simulink model "EV_Backward_Baseline"  (R2024b)
settings: Solver=FixedStepDiscrete  StartTime=EV_start  StopTime=EV_stop  FixedStep=EV_dt  RelTol=1e-3
values from neighbouring files (symbols this model uses):
  degradation_Crate = [0 0.5 1 2 3 4]    [init_ev_backward.m]    (also in initialize_model.m)
  degradation_rate = degradation_scale * [0 1 1.2 1.8 2.8 4.0]    [init_ev_backward.m]    (also in initialize_model.m = degradation_scale*degradation_relative_loss)
  ecvt_final_efficiency = EV_drive_eta    (= 0.96)    [init_ev_backward.m]    (also in initialize_model.m)
  ecvt_final_ratio = EV_final    (= 3)    [init_ev_backward.m]    (also in initialize_model.m)
  ecvt_parameters = [N_s N_r ecvt_motor1_Tmax ecvt_motor2_Tmax      ecvt_motor1_Pmax ecvt_motor2_Pmax motor1_wmax motor2_wmax      EV_motor_eta EV_regen_eta motor1_regen_fraction motor2_regen_fraction]    [init_ev_backward.m]    (also in initialize_model.m = [ecvt_parameters ecvt_strategy EV_voltage EV_resistance     )
  EV_Ah0 = 0    [initialize_model.m]
  EV_area = 2.2    [init_ev_backward.m]    (also in initialize_model.m)
  EV_capacity_Ah = 150    [init_ev_backward.m]    (also in initialize_model.m)
  EV_Cd = 0.29    [init_ev_backward.m]    (also in initialize_model.m)
  EV_Crr = 0.010    (= 0.01)    [init_ev_backward.m]    (also in initialize_model.m)
  EV_drive_eta = 0.96    [init_ev_backward.m]    (also in initialize_model.m)
  EV_dt = 0.1    [init_ev_backward.m]    (also in initialize_model.m)
  EV_final = 3    [init_ev_backward.m]    (also in initialize_model.m)
  EV_g = 9.81    [init_ev_backward.m]    (also in initialize_model.m)
  EV_gear = 3    [init_ev_backward.m]    (also in initialize_model.m)
  EV_grade = 0    [init_ev_backward.m]    (also in initialize_model.m)
  EV_mass = 1800    [init_ev_backward.m]    (also in initialize_model.m)
  EV_motor_eta = 0.92    [init_ev_backward.m]    (also in initialize_model.m)
  EV_radius = 0.31    [init_ev_backward.m]    (also in initialize_model.m)
  EV_regen_eta = 0.85    [init_ev_backward.m]    (also in initialize_model.m)
  EV_resistance = 0.08    [init_ev_backward.m]    (also in initialize_model.m)
  EV_rho = 1.225    [init_ev_backward.m]    (also in initialize_model.m)
  EV_SOC0 = 0.80    (= 0.8)    [init_ev_backward.m]    (also in initialize_model.m = 0.35)
  EV_SOH0 = 1.0    (= 1)    [init_ev_backward.m]    (also in initialize_model.m)
  EV_SOH_max = 1    [initialize_model.m]
  EV_SOH_min = 0    [initialize_model.m]
  EV_v0 = EV_speed(1)    [init_ev_backward.m]    (also in initialize_model.m)
  EV_voltage = 360    [init_ev_backward.m]    (also in initialize_model.m)
undefined symbols (not defined in the file or in its folder): DiscIntNeverNeededParam, ecvt_electrical_power, ecvt_operating_point
settings Model: Creator=menda  LastModifiedBy=menda

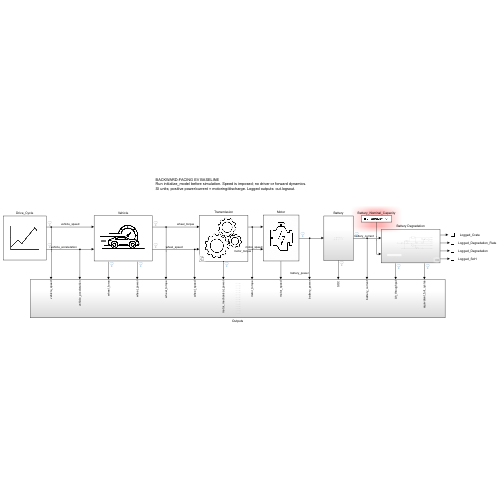
[thumbnail: Simulink's stored preview of the top-level diagram]
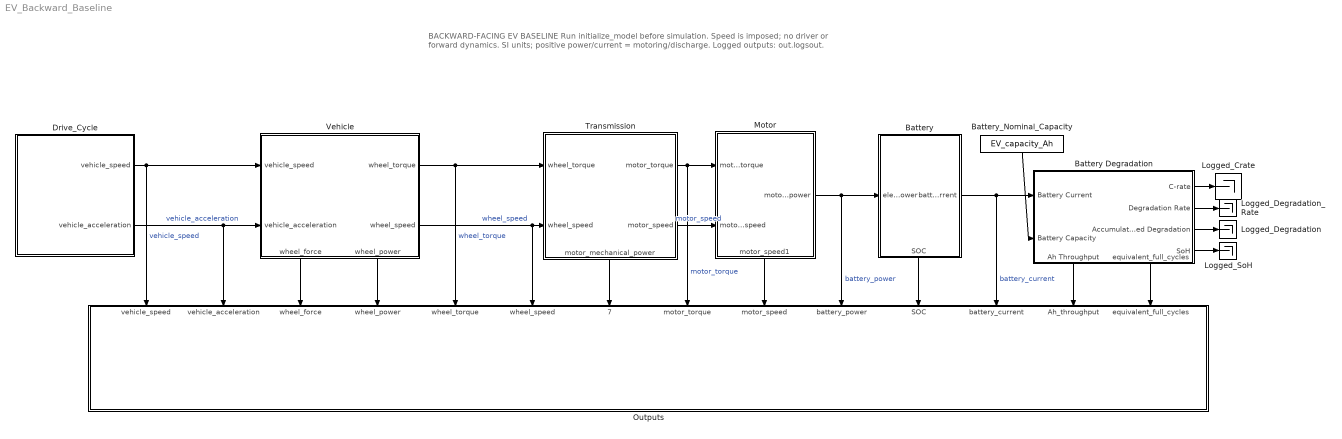
== system EV_Backward_Baseline ==
  note: BACKWARD-FACING EV BASELINE
      | Run initialize_model before simulation. Speed is imposed; no driver or forward dynamics.
      | SI units; positive power/current = motoring/discharge. Logged outputs: out.logsout.
  Battery : Subsystem  Description=Pbat=(Voc-R*I)*I; I=2*Pbat/(Voc+sqrt(Voc^2-4*R*Pbat)); dSOC/dt=-I/(3600*capacity_Ah). Positive I discharges. Assertions stop for infeasible power or SOC outside [0,1]. abs under sqrt only guards evaluation before the power assertion; it does not authorize infeasible demands.
      settings: PortSchema="{\"entries\":[{\"content\":{\"sides\":[{\"content\":{\"connectorIds\":[\"In1\"]},\"type\":\"ConnectorPlacement.EquallySpacedRectSide\",\"uuid\":\"e30f2f7f-bb89-4748-9a65-d09dfa466cc4\"},{\"content\":{\"connectorIds\":[\"Out1\"],\"side\":\"RIGHT\"},\"type\":\"ConnectorPlacement.EquallySpacedRectSide\",\"uuid\":\"7aa5349f-4bb4-43b6-83e0-f5db2de7542c\"},{\"content\":{\"side\":\"TOP\"},\"type\":\"ConnectorPlacement.EquallySpacedRectSide\",\"uuid\":\"10c9eaa9-2802-435c-9c7b-7eaef7f59c40\"},{\"content\":{\"connectorIds\":[\"Out2\"],\"side\":\"BOTTOM\"},\"type\":\"ConnectorPlacement.EquallySpacedRectSide\",\"uuid\":\"ef51e7df-83e2-4289-b7c3-b47825779f33\"}]},\"type\":\"ConnectorPlacement.EquallySpacedConnector\",\"uuid\":\"367388d2-e83d-4c8a-b099-5ce472d0570c\"}],\"packageUris\":[\"http://schema.mathworks.com/mf0/Connector/R2020b\"],\"version\":\"1.0\"}"
  Battery Degradation : Subsystem  Description=C=abs(I)/Qnom; k=f(C) [1/Ah], linear with endpoint clipping. dD/dt=k*abs(I)/3600 [1/s]; D0=1-EV_SOH0. SoH=sat(1-D,0,1). No feedback to SOC or capacity.
      settings: PortSchema="{\"entries\":[{\"content\":{\"sides\":[{\"content\":{\"connectorIds\":[\"In1\",\"In2\"]},\"type\":\"ConnectorPlacement.EquallySpacedRectSide\",\"uuid\":\"b05f624b-af73-4004-9694-629fd8fb527f\"},{\"content\":{\"connectorIds\":[\"Out1\",\"Out2\",\"Out3\",\"Out4\"],\"side\":\"RIGHT\"},\"type\":\"ConnectorPlacement.EquallySpacedRectSide\",\"uuid\":\"830d9b11-fa0e-4f63-a09e-821a7b3aefa4\"},{\"content\":{\"side\":\"TOP\"},\"type\":\"ConnectorPlacement.EquallySpacedRectSide\",\"uuid\":\"ac9d2d09-daf1-45c6-b99a-e7004515f525\"},{\"content\":{\"connectorIds\":[\"Out5\",\"Out6\"],\"side\":\"BOTTOM\"},\"type\":\"ConnectorPlacement.EquallySpacedRectSide\",\"uuid\":\"9e730963-03db-478a-aca3-248f9a9dc559\"}]},\"type\":\"ConnectorPlacement.EquallySpacedConnector\",\"uuid\":\"6a4c7b58-1cfe-457b-b589-490fcd40ae9b\"}],\"packageUris\":[\"http://schema.mathworks.com/mf0/Connector/R2020b\"],\"version\":\"1.0\"}"
  Battery_Nominal_Capacity : Constant  Value=EV_capacity_Ah
  Drive_Cycle : Subsystem  Description=Prescribed sampled speed [m/s]. a[k]=(v[k]-v[k-1])/EV_dt [m/s^2]. Initial acceleration is zero.
      mask Display: image('images/speedProfile.png');
  Logged_Crate : Terminator
  Logged_Degradation : Terminator
  Logged_Degradation_Rate : Terminator
  Logged_SoH : Terminator
  Motor : Subsystem  Description=Pmech=T*omega; Pelec=Pmech/eta_motor when Pmech>=0, otherwise Pmech*eta_regen. Positive means motoring. Torque and speed are imposed by Transmission and logged at its outputs.
      settings: PortSchema="{\"entries\":[{\"content\":{\"sides\":[{\"content\":{\"connectorIds\":[\"In1\",\"In2\"]},\"type\":\"ConnectorPlacement.EquallySpacedRectSide\",\"uuid\":\"49c52859-d992-4436-ae70-9d5acb989b00\"},{\"content\":{\"connectorIds\":[\"Out1\"],\"side\":\"RIGHT\"},\"type\":\"ConnectorPlacement.EquallySpacedRectSide\",\"uuid\":\"a77a678a-5372-480a-805a-36d1e2fecae4\"},{\"content\":{\"side\":\"TOP\"},\"type\":\"ConnectorPlacement.EquallySpacedRectSide\",\"uuid\":\"187b8372-9e3a-4a7e-b220-549ea4957a3e\"},{\"content\":{\"connectorIds\":[\"Out2\"],\"side\":\"BOTTOM\"},\"type\":\"ConnectorPlacement.EquallySpacedRectSide\",\"uuid\":\"92a127f9-6f51-4bd3-badd-4b9089e059fd\"}]},\"type\":\"ConnectorPlacement.EquallySpacedConnector\",\"uuid\":\"4c2fc29c-556e-423a-96d4-0ac59323ac06\"}],\"packageUris\":[\"http://schema.mathworks.com/mf0/Connector/R2020b\"],\"version\":\"1.0\"}"
      mask Display: image('images/engine2.jpg');
  Outputs : Subsystem
  Transmission : Subsystem  Description=Variant powertrain topology. EV_topology=1 selects single motor, fixed gear and differential. Match port names in future choices.  Variant=on
      settings: PortSchema="{\"entries\":[{\"content\":{\"sides\":[{\"content\":{\"connectorIds\":[\"In1\",\"In2\"]},\"type\":\"ConnectorPlacement.EquallySpacedRectSide\",\"uuid\":\"907b9752-0237-4bf5-b44c-0c58cc455c3d\"},{\"content\":{\"connectorIds\":[\"Out1\",\"Out2\"],\"side\":\"RIGHT\"},\"type\":\"ConnectorPlacement.EquallySpacedRectSide\",\"uuid\":\"60baf348-a017-4c22-82d9-e85b283ea42b\"},{\"content\":{\"side\":\"TOP\"},\"type\":\"ConnectorPlacement.EquallySpacedRectSide\",\"uuid\":\"1e1150ea-72dd-48d2-abb5-aeef63cf3690\"},{\"content\":{\"connectorIds\":[\"Out3\"],\"side\":\"BOTTOM\"},\"type\":\"ConnectorPlacement.EquallySpacedRectSide\",\"uuid\":\"c29cbbf6-43d5-4701-ab56-40ad23203659\"}]},\"type\":\"ConnectorPlacement.EquallySpacedConnector\",\"uuid\":\"b8b54c79-4f22-4cf5-bff2-51665ec3e128\"}],\"packageUris\":[\"http://schema.mathworks.com/mf0/Connector/R2020b\"],\"version\":\"1.0\"}"
      mask Display: image('images/Gearbox.png');
  Vehicle : Subsystem  Description=F=m*a+0.5*rho*Cd*A*v*abs(v)+Crr*m*g*cos(grade)*sign(v)+m*g*sin(grade). T=F*r; omega=v/r; P=T*omega. SI units.
      settings: PortSchema="{\"entries\":[{\"content\":{\"sides\":[{\"content\":{\"connectorIds\":[\"In1\",\"In2\"]},\"type\":\"ConnectorPlacement.EquallySpacedRectSide\",\"uuid\":\"b24511cd-7d01-487c-854b-51850ccf7238\"},{\"content\":{\"connectorIds\":[\"Out1\",\"Out2\"],\"side\":\"RIGHT\"},\"type\":\"ConnectorPlacement.EquallySpacedRectSide\",\"uuid\":\"d60f9975-1cca-4220-8342-8a527ad4bc8f\"},{\"content\":{\"side\":\"TOP\"},\"type\":\"ConnectorPlacement.EquallySpacedRectSide\",\"uuid\":\"ffffd604-d748-4b68-bba9-21435e47b16e\"},{\"content\":{\"connectorIds\":[\"Out3\",\"Out4\"],\"side\":\"BOTTOM\"},\"type\":\"ConnectorPlacement.EquallySpacedRectSide\",\"uuid\":\"c964c0b3-1bf1-4a71-99c2-52acac1d6e4c\"}]},\"type\":\"ConnectorPlacement.EquallySpacedConnector\",\"uuid\":\"2b03c9da-f0d0-45d9-9588-bb20003291c2\"}],\"packageUris\":[\"http://schema.mathworks.com/mf0/Connector/R2020b\"],\"version\":\"1.0\"}"
      mask Display: image('images/Dynamics.png');
  wires:
  Vehicle/1(wheel_torque) -> Outputs/5(wheel_torque), Transmission/1(wheel_torque)  "wheel_torque"
  Drive_Cycle/1(vehicle_speed) -> Outputs/1(vehicle_speed), Vehicle/1(vehicle_speed)  "vehicle_speed"
  Drive_Cycle/2(vehicle_acceleration) -> Outputs/2(vehicle_acceleration), Vehicle/2(vehicle_acceleration)  "vehicle_acceleration"
  Vehicle/2(wheel_speed) -> Outputs/6(wheel_speed), Transmission/2(wheel_speed)  "wheel_speed"
  Battery/1(battery_current) -> Outputs/12(battery_current), Battery Degradation/1(Battery Current)  "battery_current"
  Vehicle/3(wheel_force) -> Outputs/3(wheel_force)
  Vehicle/4(wheel_power) -> Outputs/4(wheel_power)
  Motor/1(motor_electrical_power) -> Outputs/10(battery_power), Battery/1(electrical_power)  "battery_power"
  Battery/2(SOC) -> Outputs/11(SOC)
  Battery Degradation/5(Ah Throughput) -> Outputs/13(Ah_throughput)
  Battery Degradation/6(equivalent_full_cycles) -> Outputs/14(equivalent_full_cycles)
  Transmission/3(motor_mechanical_power) -> Outputs/7(motor_mechanical_power)
  Transmission/1(motor_torque) -> Outputs/8(motor_torque), Motor/1(motor_torque)  "motor_torque"
  Transmission/2(motor_speed) -> Motor/2(motor_speed)  "motor_speed"
  Battery_Nominal_Capacity/1 -> Battery Degradation/2(Battery Capacity)
  Battery Degradation/1(C-rate) -> Logged_Crate/1
  Battery Degradation/2(Degradation Rate) -> Logged_Degradation_Rate/1
  Battery Degradation/3(Accumulated Degradation) -> Logged_Degradation/1
  Battery Degradation/4(SoH) -> Logged_SoH/1
  Motor/2(motor_speed1) -> Outputs/9(motor_speed)

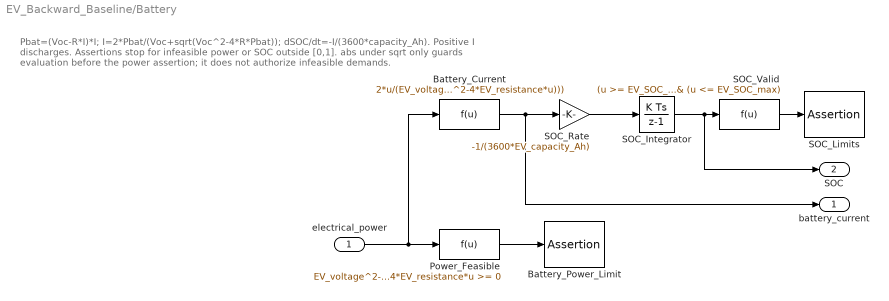
== system EV_Backward_Baseline/Battery ==
  note: Pbat=(Voc-R*I)*I; I=2*Pbat/(Voc+sqrt(Voc^2-4*R*Pbat)); dSOC/dt=-I/(3600*capacity_Ah). Positive I discharges. Assertions stop for infeasible power or SOC outside [0,1]. abs under sqrt only guards evaluation before the power assertion; it does not authorize infeasible demands.
  electrical_power : Inport
  Battery_Current : Fcn  Expr=2*u/(EV_voltage+sqrt(abs(EV_voltage^2-4*EV_resistance*u)))
  Battery_Power_Limit : Assertion
  Power_Feasible : Fcn  Expr=EV_voltage^2-4*EV_resistance*u >= 0
  SOC_Integrator : DiscreteIntegrator  InitialCondition=EV_SOC0  SampleTime=EV_dt  ICPrevOutput=DiscIntNeverNeededParam  ICPrevScaledInput=DiscIntNeverNeededParam
  SOC_Limits : Assertion
  SOC_Rate : Gain  Gain=-1/(3600*EV_capacity_Ah)
  SOC_Valid : Fcn  Expr=(u >= EV_SOC_min) && (u <= EV_SOC_max)
  battery_current : Outport
  SOC : Outport  Port=2
  wires:
  SOC_Valid/1 -> SOC_Limits/1
  SOC_Integrator/1 -> SOC/1, SOC_Valid/1
  SOC_Rate/1 -> SOC_Integrator/1
  Battery_Current/1 -> battery_current/1, SOC_Rate/1
  Power_Feasible/1 -> Battery_Power_Limit/1
  electrical_power/1 -> Battery_Current/1, Power_Feasible/1

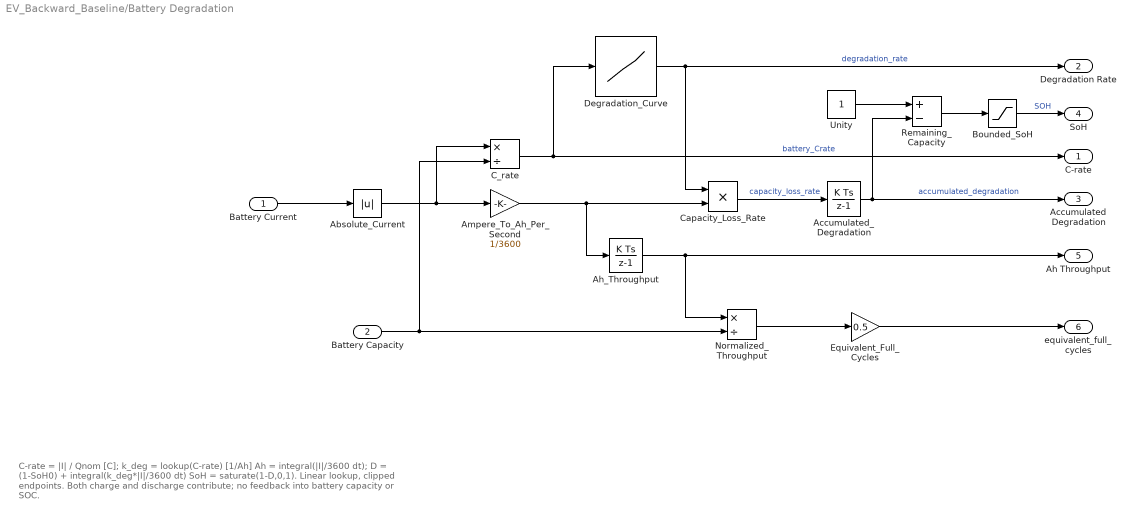
== system EV_Backward_Baseline/Battery Degradation ==
  note: C-rate = |I| / Qnom [C]; k_deg = lookup(C-rate) [1/Ah]
      | Ah = integral(|I|/3600 dt); D = (1-SoH0) + integral(k_deg*|I|/3600 dt)
      | SoH = saturate(1-D,0,1). Linear lookup, clipped endpoints.
      | Both charge and discharge contribute; no feedback into battery capacity or SOC.
  Battery Current : Inport
  Battery Capacity : Inport  Port=2
  Absolute_Current : Abs  SaturateOnIntegerOverflow=off
  Accumulated_Degradation : DiscreteIntegrator  InitialCondition=1-EV_SOH0  SampleTime=EV_dt  ICPrevOutput=DiscIntNeverNeededParam  ICPrevScaledInput=DiscIntNeverNeededParam
  Ah_Throughput : DiscreteIntegrator  InitialCondition=EV_Ah0  SampleTime=EV_dt  ICPrevOutput=DiscIntNeverNeededParam  ICPrevScaledInput=DiscIntNeverNeededParam
  Ampere_To_Ah_Per_Second : Gain  Gain=1/3600
  Bounded_SoH : Saturate  UpperLimit=EV_SOH_max  LowerLimit=EV_SOH_min
  C_rate : Product  Inputs=*/
  Capacity_Loss_Rate : Product  Inputs=**
  Degradation_Curve : Lookup_n-D  NumberOfTableDimensions=1  BreakpointsForDimension1=degradation_Crate  Table=degradation_rate  ExtrapMethod=Clip  InternalRulePriority=Speed  RndMeth=Simplest
  Equivalent_Full_Cycles : Gain  Gain=0.5
  Normalized_Throughput : Product  Inputs=*/
  Remaining_Capacity : Sum  Inputs=+-
  Unity : Constant
  C-rate : Outport
  Degradation Rate : Outport  Port=2
  Accumulated Degradation : Outport  Port=3
  SoH : Outport  Port=4
  Ah Throughput : Outport  Port=5
  equivalent_full_cycles : Outport  Port=6
  wires:
  Normalized_Throughput/1 -> Equivalent_Full_Cycles/1
  Bounded_SoH/1 -> SoH/1  "SOH"
  Remaining_Capacity/1 -> Bounded_SoH/1
  Unity/1 -> Remaining_Capacity/1
  Accumulated_Degradation/1 -> Accumulated Degradation/1, Remaining_Capacity/2  "accumulated_degradation"
  Capacity_Loss_Rate/1 -> Accumulated_Degradation/1  "capacity_loss_rate"
  Degradation_Curve/1 -> Capacity_Loss_Rate/1, Degradation Rate/1  "degradation_rate"
  C_rate/1 -> Degradation_Curve/1, C-rate/1  "battery_Crate"
  Battery Capacity/1 -> C_rate/2, Normalized_Throughput/2
  Absolute_Current/1 -> C_rate/1, Ampere_To_Ah_Per_Second/1
  Ampere_To_Ah_Per_Second/1 -> Ah_Throughput/1, Capacity_Loss_Rate/2
  Ah_Throughput/1 -> Ah Throughput/1, Normalized_Throughput/1
  Equivalent_Full_Cycles/1 -> equivalent_full_cycles/1
  Battery Current/1 -> Absolute_Current/1

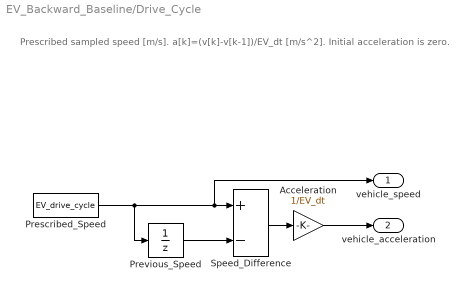
== system EV_Backward_Baseline/Drive_Cycle ==
  note: Prescribed sampled speed [m/s]. a[k]=(v[k]-v[k-1])/EV_dt [m/s^2]. Initial acceleration is zero.
  Acceleration : Gain  Gain=1/EV_dt
  Prescribed_Speed : FromWorkspace  VariableName=EV_drive_cycle  SampleTime=EV_dt
  Previous_Speed : UnitDelay  InitialCondition=EV_v0  SampleTime=EV_dt  HasFrameUpgradeWarning=on
  Speed_Difference : Sum  Inputs=+-
  vehicle_speed : Outport
  vehicle_acceleration : Outport  Port=2
  wires:
  Acceleration/1 -> vehicle_acceleration/1
  Speed_Difference/1 -> Acceleration/1
  Previous_Speed/1 -> Speed_Difference/2
  Prescribed_Speed/1 -> vehicle_speed/1, Speed_Difference/1, Previous_Speed/1

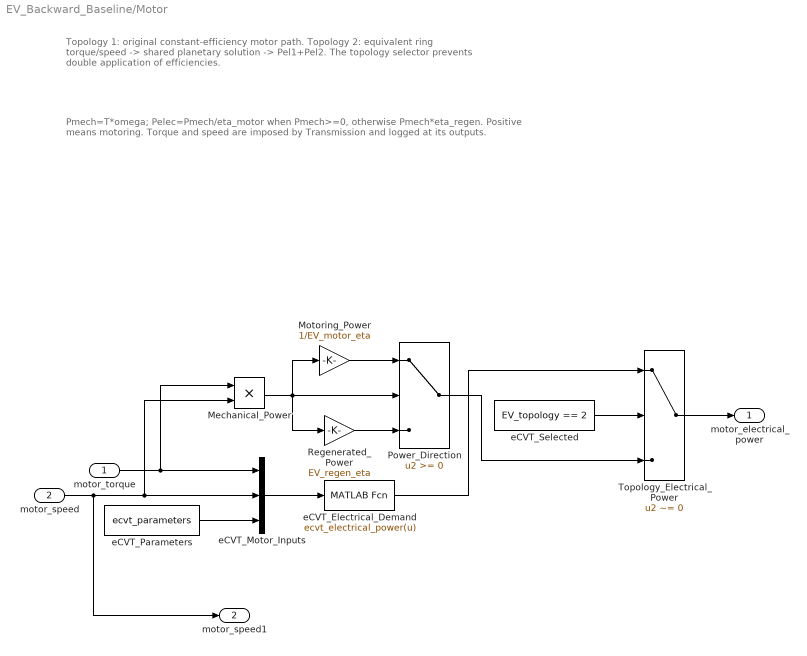
== system EV_Backward_Baseline/Motor ==
  note: Pmech=T*omega; Pelec=Pmech/eta_motor when Pmech>=0, otherwise Pmech*eta_regen. Positive means motoring. Torque and speed are imposed by Transmission and logged at its outputs.
  note: Topology 1: original constant-efficiency motor path.
      | Topology 2: equivalent ring torque/speed -> shared planetary solution -> Pel1+Pel2.
      | The topology selector prevents double application of efficiencies.
  motor_torque : Inport
  motor_speed : Inport  Port=2
  Mechanical_Power : Product
  Motoring_Power : Gain  Gain=1/EV_motor_eta
  Power_Direction : Switch  SaturateOnIntegerOverflow=off  InputSameDT=off
  Regenerated_Power : Gain  Gain=EV_regen_eta
  Topology_Electrical_Power : Switch  Criteria=u2 ~= 0  SaturateOnIntegerOverflow=off  InputSameDT=off
  eCVT_Electrical_Demand : MATLABFcn  MATLABFcn=ecvt_electrical_power(u)  OutputDimensions=1
  eCVT_Motor_Inputs : Mux  Inputs=3
  eCVT_Parameters : Constant  Value=ecvt_parameters
  eCVT_Selected : Constant  Value=EV_topology == 2
  motor_electrical_power : Outport
  motor_speed1 : Outport  Port=2
  wires:
  motor_torque/1 -> Mechanical_Power/1, eCVT_Motor_Inputs/1
  motor_speed/1 -> motor_speed1/1, eCVT_Motor_Inputs/2, Mechanical_Power/2
  Mechanical_Power/1 -> Regenerated_Power/1, Motoring_Power/1, Power_Direction/2
  Motoring_Power/1 -> Power_Direction/1
  Regenerated_Power/1 -> Power_Direction/3
  Topology_Electrical_Power/1 -> motor_electrical_power/1
  eCVT_Selected/1 -> Topology_Electrical_Power/2
  eCVT_Electrical_Demand/1 -> Topology_Electrical_Power/1
  Power_Direction/1 -> Topology_Electrical_Power/3
  eCVT_Parameters/1 -> eCVT_Motor_Inputs/3
  eCVT_Motor_Inputs/1 -> eCVT_Electrical_Demand/1

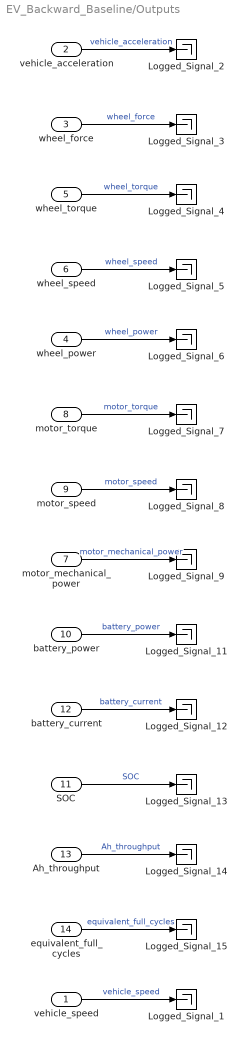
== system EV_Backward_Baseline/Outputs ==
  vehicle_speed : Inport
  vehicle_acceleration : Inport  Port=2
  wheel_force : Inport  Port=3
  wheel_power : Inport  Port=4
  wheel_torque : Inport  Port=5
  wheel_speed : Inport  Port=6
  motor_mechanical_power : Inport  Port=7
  motor_torque : Inport  Port=8
  motor_speed : Inport  Port=9
  battery_power : Inport  Port=10
  SOC : Inport  Port=11
  battery_current : Inport  Port=12
  Ah_throughput : Inport  Port=13
  equivalent_full_cycles : Inport  Port=14
  Logged_Signal_{1..9,11..15} (14 alike) : Terminator
  wires:
  vehicle_speed/1 -> Logged_Signal_1/1  "vehicle_speed"
  vehicle_acceleration/1 -> Logged_Signal_2/1  "vehicle_acceleration"
  wheel_force/1 -> Logged_Signal_3/1  "wheel_force"
  wheel_torque/1 -> Logged_Signal_4/1  "wheel_torque"
  wheel_speed/1 -> Logged_Signal_5/1  "wheel_speed"
  wheel_power/1 -> Logged_Signal_6/1  "wheel_power"
  motor_torque/1 -> Logged_Signal_7/1  "motor_torque"
  motor_speed/1 -> Logged_Signal_8/1  "motor_speed"
  motor_mechanical_power/1 -> Logged_Signal_9/1  "motor_mechanical_power"
  battery_power/1 -> Logged_Signal_11/1  "battery_power"
  battery_current/1 -> Logged_Signal_12/1  "battery_current"
  SOC/1 -> Logged_Signal_13/1  "SOC"
  Ah_throughput/1 -> Logged_Signal_14/1  "Ah_throughput"
  equivalent_full_cycles/1 -> Logged_Signal_15/1  "equivalent_full_cycles"

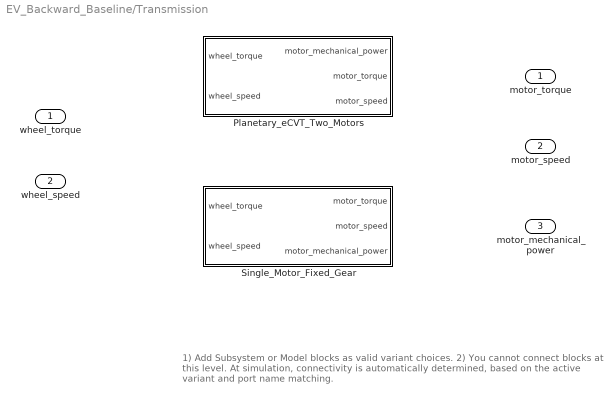
== system EV_Backward_Baseline/Transmission ==
  note: 1) Add Subsystem or Model blocks as valid variant choices.
      | 2) You cannot connect blocks at this level. At simulation, connectivity is automatically
      | determined, based on the active variant and port name matching.
  wheel_torque : Inport
  wheel_speed : Inport  Port=2
  Planetary_eCVT_Two_Motors : Subsystem  Description=Ideal planetary: M1 sun, M2 carrier, output ring. Scalar outputs are equivalent ring mechanical power/torque/speed. See README_eCVT.md.  VariantControl=EV_topology == 2
  Single_Motor_Fixed_Gear : Subsystem  Description=ratio=EV_gear*EV_final; omega_m=ratio*omega_w. T_m=T_w/(ratio*eta_d) for motoring, T_w*eta_d/ratio for regeneration. Combined gear/differential losses; no shaft inertia.  VariantControl=EV_topology == 1
  motor_torque : Outport
  motor_speed : Outport  Port=2
  motor_mechanical_power : Outport  Port=3

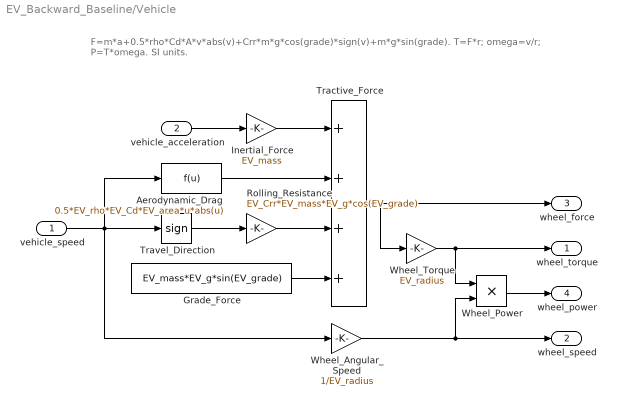
== system EV_Backward_Baseline/Vehicle ==
  note: F=m*a+0.5*rho*Cd*A*v*abs(v)+Crr*m*g*cos(grade)*sign(v)+m*g*sin(grade). T=F*r; omega=v/r; P=T*omega. SI units.
  vehicle_speed : Inport
  vehicle_acceleration : Inport  Port=2
  Aerodynamic_Drag : Fcn  Expr=0.5*EV_rho*EV_Cd*EV_area*u*abs(u)
  Grade_Force : Constant  Value=EV_mass*EV_g*sin(EV_grade)
  Inertial_Force : Gain  Gain=EV_mass
  Rolling_Resistance : Gain  Gain=EV_Crr*EV_mass*EV_g*cos(EV_grade)
  Tractive_Force : Sum  Inputs=++++
  Travel_Direction : Signum
  Wheel_Angular_Speed : Gain  Gain=1/EV_radius
  Wheel_Power : Product
  Wheel_Torque : Gain  Gain=EV_radius
  wheel_torque : Outport
  wheel_speed : Outport  Port=2
  wheel_force : Outport  Port=3
  wheel_power : Outport  Port=4
  wires:
  Wheel_Power/1 -> wheel_power/1
  Wheel_Angular_Speed/1 -> wheel_speed/1, Wheel_Power/2
  Wheel_Torque/1 -> Wheel_Power/1, wheel_torque/1
  Tractive_Force/1 -> wheel_force/1, Wheel_Torque/1
  Grade_Force/1 -> Tractive_Force/4
  Rolling_Resistance/1 -> Tractive_Force/3
  Aerodynamic_Drag/1 -> Tractive_Force/2
  Inertial_Force/1 -> Tractive_Force/1
  Travel_Direction/1 -> Rolling_Resistance/1
  vehicle_acceleration/1 -> Inertial_Force/1
  vehicle_speed/1 -> Wheel_Angular_Speed/1, Aerodynamic_Drag/1, Travel_Direction/1

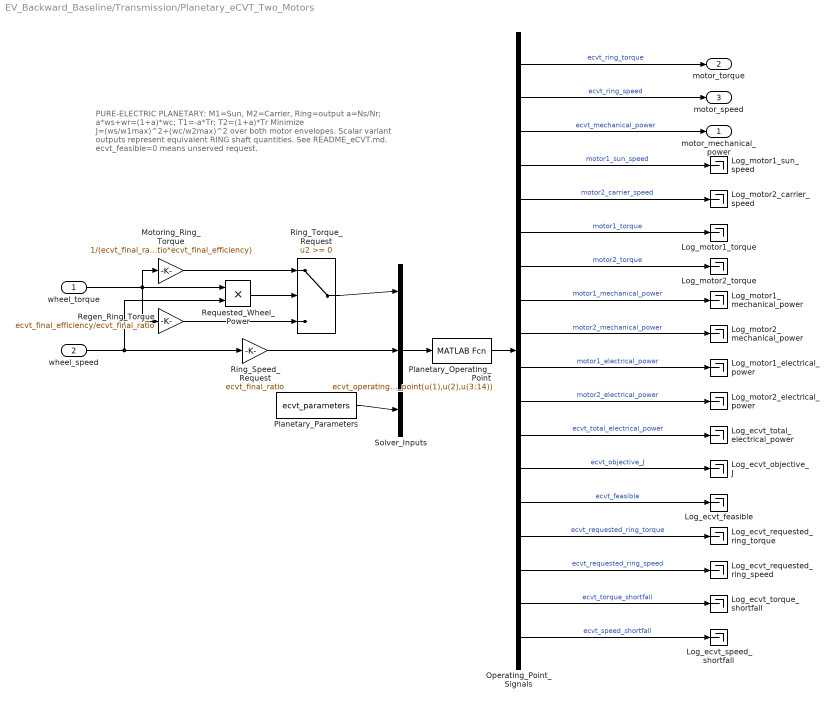
== system EV_Backward_Baseline/Transmission/Planetary_eCVT_Two_Motors ==
  note: PURE-ELECTRIC PLANETARY: M1=Sun, M2=Carrier, Ring=output
      | a=Ns/Nr; a*ws+wr=(1+a)*wc; T1=-a*Tr; T2=(1+a)*Tr
      | Minimize J=(ws/w1max)^2+(wc/w2max)^2 over both motor envelopes.
      | Scalar variant outputs represent equivalent RING shaft quantities.
      | See README_eCVT.md. ecvt_feasible=0 means unserved request.
  wheel_torque : Inport
  wheel_speed : Inport  Port=2
  Log_ecvt_feasible : Terminator
  Log_ecvt_objective_J : Terminator
  Log_ecvt_requested_ring_speed : Terminator
  Log_ecvt_requested_ring_torque : Terminator
  Log_ecvt_speed_shortfall : Terminator
  Log_ecvt_torque_shortfall : Terminator
  Log_ecvt_total_electrical_power : Terminator
  Log_motor1_electrical_power : Terminator
  Log_motor1_mechanical_power : Terminator
  Log_motor1_sun_speed : Terminator
  Log_motor1_torque : Terminator
  Log_motor2_carrier_speed : Terminator
  Log_motor2_electrical_power : Terminator
  Log_motor2_mechanical_power : Terminator
  Log_motor2_torque : Terminator
  Motoring_Ring_Torque : Gain  Gain=1/(ecvt_final_ratio*ecvt_final_efficiency)
  Operating_Point_Signals : Demux  Outputs=18
  Planetary_Operating_Point : MATLABFcn  MATLABFcn=ecvt_operating_point(u(1),u(2),u(3:14))  OutputDimensions=18
  Planetary_Parameters : Constant  Value=ecvt_parameters
  Regen_Ring_Torque : Gain  Gain=ecvt_final_efficiency/ecvt_final_ratio
  Requested_Wheel_Power : Product  Inputs=**
  Ring_Speed_Request : Gain  Gain=ecvt_final_ratio
  Ring_Torque_Request : Switch  SaturateOnIntegerOverflow=off  InputSameDT=off
  Solver_Inputs : Mux  Inputs=3
  motor_mechanical_power : Outport
  motor_torque : Outport  Port=2
  motor_speed : Outport  Port=3
  wires:
  wheel_torque/1 -> Regen_Ring_Torque/1, Motoring_Ring_Torque/1, Requested_Wheel_Power/1
  wheel_speed/1 -> Requested_Wheel_Power/2, Ring_Speed_Request/1
  Motoring_Ring_Torque/1 -> Ring_Torque_Request/1
  Requested_Wheel_Power/1 -> Ring_Torque_Request/2
  Regen_Ring_Torque/1 -> Ring_Torque_Request/3
  Operating_Point_Signals/4 -> Log_motor1_sun_speed/1  "motor1_sun_speed"
  Operating_Point_Signals/5 -> Log_motor2_carrier_speed/1  "motor2_carrier_speed"
  Operating_Point_Signals/6 -> Log_motor1_torque/1  "motor1_torque"
  Operating_Point_Signals/7 -> Log_motor2_torque/1  "motor2_torque"
  Operating_Point_Signals/8 -> Log_motor1_mechanical_power/1  "motor1_mechanical_power"
  Operating_Point_Signals/9 -> Log_motor2_mechanical_power/1  "motor2_mechanical_power"
  Operating_Point_Signals/10 -> Log_motor1_electrical_power/1  "motor1_electrical_power"
  Operating_Point_Signals/11 -> Log_motor2_electrical_power/1  "motor2_electrical_power"
  Operating_Point_Signals/12 -> Log_ecvt_total_electrical_power/1  "ecvt_total_electrical_power"
  Operating_Point_Signals/13 -> Log_ecvt_objective_J/1  "ecvt_objective_J"
  Operating_Point_Signals/14 -> Log_ecvt_feasible/1  "ecvt_feasible"
  Operating_Point_Signals/15 -> Log_ecvt_requested_ring_torque/1  "ecvt_requested_ring_torque"
  Operating_Point_Signals/16 -> Log_ecvt_requested_ring_speed/1  "ecvt_requested_ring_speed"
  Operating_Point_Signals/17 -> Log_ecvt_torque_shortfall/1  "ecvt_torque_shortfall"
  Operating_Point_Signals/18 -> Log_ecvt_speed_shortfall/1  "ecvt_speed_shortfall"
  Operating_Point_Signals/3 -> motor_mechanical_power/1  "ecvt_mechanical_power"
  Operating_Point_Signals/2 -> motor_speed/1  "ecvt_ring_speed"
  Operating_Point_Signals/1 -> motor_torque/1  "ecvt_ring_torque"
  Planetary_Operating_Point/1 -> Operating_Point_Signals/1
  Solver_Inputs/1 -> Planetary_Operating_Point/1
  Ring_Speed_Request/1 -> Solver_Inputs/2
  Ring_Torque_Request/1 -> Solver_Inputs/1
  Planetary_Parameters/1 -> Solver_Inputs/3

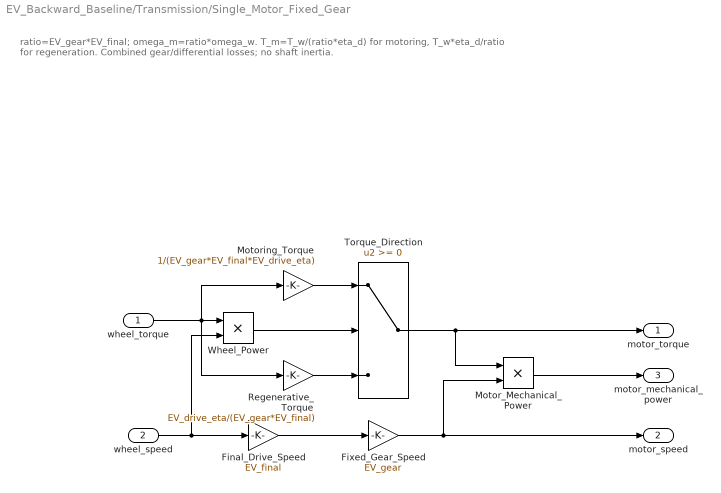
== system EV_Backward_Baseline/Transmission/Single_Motor_Fixed_Gear ==
  note: ratio=EV_gear*EV_final; omega_m=ratio*omega_w. T_m=T_w/(ratio*eta_d) for motoring, T_w*eta_d/ratio for regeneration. Combined gear/differential losses; no shaft inertia.
  wheel_torque : Inport
  wheel_speed : Inport  Port=2
  Final_Drive_Speed : Gain  Gain=EV_final
  Fixed_Gear_Speed : Gain  Gain=EV_gear
  Motor_Mechanical_Power : Product
  Motoring_Torque : Gain  Gain=1/(EV_gear*EV_final*EV_drive_eta)
  Regenerative_Torque : Gain  Gain=EV_drive_eta/(EV_gear*EV_final)
  Torque_Direction : Switch  SaturateOnIntegerOverflow=off  InputSameDT=off
  Wheel_Power : Product
  motor_torque : Outport
  motor_speed : Outport  Port=2
  motor_mechanical_power : Outport  Port=3
  wires:
  Motor_Mechanical_Power/1 -> motor_mechanical_power/1
  Torque_Direction/1 -> motor_torque/1, Motor_Mechanical_Power/1
  Regenerative_Torque/1 -> Torque_Direction/3
  Motoring_Torque/1 -> Torque_Direction/1
  Wheel_Power/1 -> Torque_Direction/2
  wheel_torque/1 -> Motoring_Torque/1, Regenerative_Torque/1, Wheel_Power/1
  Fixed_Gear_Speed/1 -> Motor_Mechanical_Power/2, motor_speed/1
  wheel_speed/1 -> Final_Drive_Speed/1, Wheel_Power/2
  Final_Drive_Speed/1 -> Fixed_Gear_Speed/1
